simulink model "modelh_age"  (R2020b)
settings: Solver=VariableStepAuto  StartTime=0.0  StopTime=10.0  RelTol=1e-3
values from neighbouring files (symbols this model uses):
  alphaH = 1-exp(-1/d_Hj)    [parameters.m]
  alphaI = 1-exp(-d_Is)    [parameters.m]
  alphaJ = 1-exp(-1/d_J)    [parameters.m]
  gammaA = 1-exp(-1/d_Ia)    [parameters.m]
  gammaH = 1-exp(-1/d_Hr)    [parameters.m]
  gammaZ = 1-exp(-1/d_Iz)    [parameters.m]
  p_d_mu = 0.49    [parameters.m]
  p_d_sd = 0.1    [parameters.m]
  p_h = 0.055    [parameters.m]
  p_j_mu = 0.23    [parameters.m]
  p_j_sd = 0.1    [parameters.m]
  p_s_h = 0.99    [parameters.m]
  p_s_l = 0.5    [parameters.m]
  psi = 1-exp(-1/d_Ip)    [parameters.m]
  r_beta_h = 0.99    [parameters.m]
  r_beta_l = 0.4    [parameters.m]
  r_c_h = 0.5    [parameters.m]
  r_c_l = 0.01    [parameters.m]
  sigma = 1 - exp(-1/d_E)    [parameters.m]
settings Model: Creator=vikroe  LastModifiedBy=vikroe

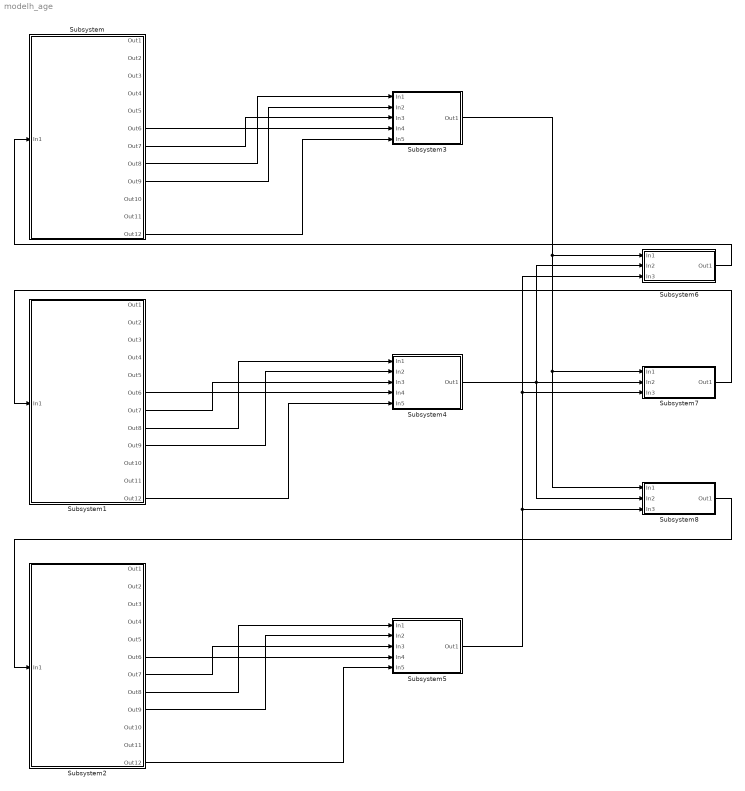
== system modelh_age ==
  Subsystem : Subsystem
  Subsystem1 : Subsystem
  Subsystem2 : Subsystem
  Subsystem3 : Subsystem
  Subsystem4 : Subsystem
  Subsystem5 : Subsystem
  Subsystem6 : Subsystem
  Subsystem7 : Subsystem
  Subsystem8 : Subsystem
  wires:
  Subsystem/12(Out12) -> Subsystem3/5(In5)
  Subsystem/8(Out8) -> Subsystem3/1(In1)
  Subsystem/9(Out9) -> Subsystem3/2(In2)
  Subsystem/7(Out7) -> Subsystem3/3(In3)
  Subsystem/6(Out6) -> Subsystem3/4(In4)
  Subsystem1/6(Out6) -> Subsystem4/4(In4)
  Subsystem1/8(Out8) -> Subsystem4/1(In1)
  Subsystem1/7(Out7) -> Subsystem4/3(In3)
  Subsystem1/9(Out9) -> Subsystem4/2(In2)
  Subsystem1/12(Out12) -> Subsystem4/5(In5)
  Subsystem2/6(Out6) -> Subsystem5/4(In4)
  Subsystem2/8(Out8) -> Subsystem5/1(In1)
  Subsystem2/7(Out7) -> Subsystem5/3(In3)
  Subsystem2/9(Out9) -> Subsystem5/2(In2)
  Subsystem2/12(Out12) -> Subsystem5/5(In5)
  Subsystem3/1(Out1) -> Subsystem6/1(In1), Subsystem7/1(In1), Subsystem8/1(In1)
  Subsystem4/1(Out1) -> Subsystem8/2(In2), Subsystem6/2(In2), Subsystem7/2(In2)
  Subsystem5/1(Out1) -> Subsystem8/3(In3), Subsystem7/3(In3), Subsystem6/3(In3)
  Subsystem6/1(Out1) -> Subsystem/1(In1)
  Subsystem7/1(Out1) -> Subsystem1/1(In1)
  Subsystem8/1(Out1) -> Subsystem2/1(In1)

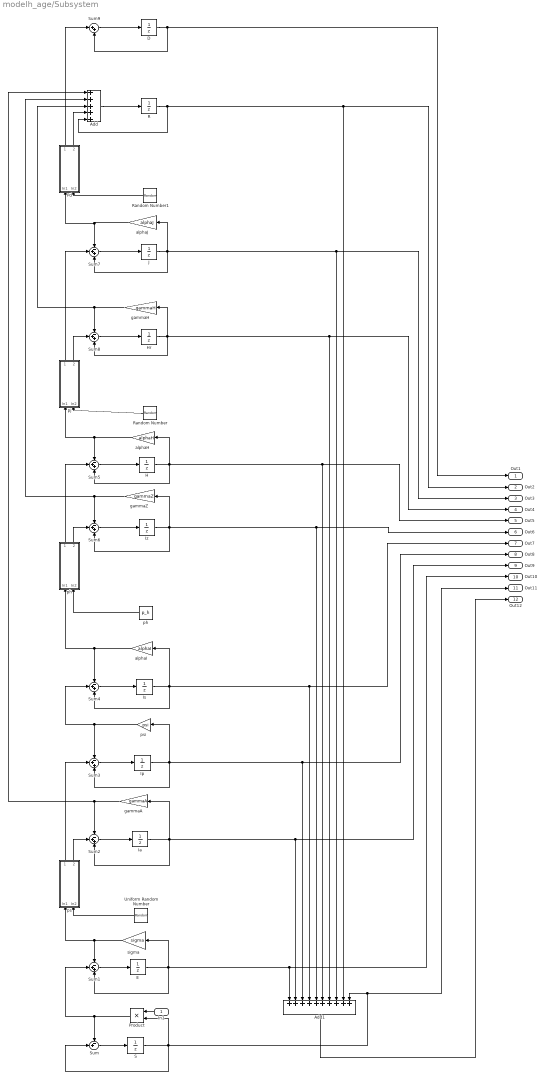
== system modelh_age/Subsystem ==
  In1 : Inport
  Add : Sum  Inputs=+++++
  Add1 : Sum  Inputs=++++++++++
  D : UnitDelay  SampleTime=-1  HasFrameUpgradeWarning=on
  E : UnitDelay  InitialCondition=10000  SampleTime=-1  HasFrameUpgradeWarning=on
  H : UnitDelay  InitialCondition=5000  SampleTime=-1  HasFrameUpgradeWarning=on
  Hr : UnitDelay  InitialCondition=5000  SampleTime=-1  HasFrameUpgradeWarning=on
  Ia : UnitDelay  InitialCondition=5000  SampleTime=-1  HasFrameUpgradeWarning=on
  Ip : UnitDelay  InitialCondition=5000  SampleTime=-1  HasFrameUpgradeWarning=on
  Is : UnitDelay  InitialCondition=5000  SampleTime=-1  HasFrameUpgradeWarning=on
  Iz : UnitDelay  InitialCondition=5000  SampleTime=-1  HasFrameUpgradeWarning=on
  J : UnitDelay  InitialCondition=5000  SampleTime=-1  HasFrameUpgradeWarning=on
  Pd : Subsystem
  Product : Product
  R : UnitDelay  InitialCondition=5000  SampleTime=-1  HasFrameUpgradeWarning=on
  Random Number : RandomNumber  Mean=p_j_mu  Variance=p_j_sd  SampleTime=0.1
  Random Number1 : RandomNumber  Mean=p_d_mu  Variance=p_d_sd  SampleTime=0.1
  S : UnitDelay  InitialCondition=5000000  SampleTime=-1  HasFrameUpgradeWarning=on
  Sum : Sum  Inputs=-+|
  Sum{1..8} (8 alike) : Sum  Inputs=-++
  Sum9 : Sum  Inputs=|++
  Uniform Random Number : UniformRandomNumber  Minimum=p_s_l  Maximum=p_s_h  SampleTime=0.1
  alphaH : Gain  Gain=alphaH
  alphaI : Gain  Gain=alphaI
  alphaJ : Gain  Gain=alphaJ
  gammaA : Gain  Gain=gammaA
  gammaH : Gain  Gain=gammaH
  gammaZ : Gain  Gain=gammaZ
  ph : Subsystem
  "ph " : Constant  Value=p_h
  pj : Subsystem
  "ps " : Subsystem
  psi : Gain  Gain=psi
  sigma : Gain  Gain=sigma
  Out1 : Outport
  Out2 : Outport  Port=2
  Out3 : Outport  Port=3
  Out4 : Outport  Port=4
  Out5 : Outport  Port=5
  Out6 : Outport  Port=6
  Out7 : Outport  Port=7
  Out8 : Outport  Port=8
  Out9 : Outport  Port=9
  Out10 : Outport  Port=10
  Out11 : Outport  Port=11
  Out12 : Outport  Port=12
  wires:
  Sum5/1 -> H/1
  alphaH/1 -> pj/1(In1), Sum5/1
  gammaH/1 -> Sum8/1, Add/3
  "ph "/1 -> ph/2(In2)
  "ps "/1(Out1) -> Sum3/2
  Uniform Random Number/1 -> "ps "/2(In2)
  J/1 -> Out3/1, Add1/8, alphaJ/1, Sum7/3
  ph/1(Out1) -> Sum5/2
  Iz/1 -> Out6/1, Add1/5, gammaZ/1, Sum6/3
  Ip/1 -> Out8/1, Add1/3, psi/1, Sum3/3
  alphaJ/1 -> Pd/1(In1), Sum7/1
  psi/1 -> Sum4/2, Sum3/1
  Ia/1 -> Out9/1, Add1/2, gammaA/1, Sum2/3
  Sum8/1 -> Hr/1
  Sum6/1 -> Iz/1
  Hr/1 -> Out4/1, Add1/7, gammaH/1, Sum8/3
  gammaA/1 -> Sum2/1, Add/1
  Sum4/1 -> Is/1
  D/1 -> Out1/1, Sum9/2
  pj/1(Out1) -> Sum7/2
  Add1/1 -> Out12/1
  Sum1/1 -> E/1
  R/1 -> Out2/1, Add1/9, Add/5
  E/1 -> Out10/1, Add1/1, sigma/1, Sum1/3
  Sum2/1 -> Ia/1
  pj/2(Out2) -> Sum8/2
  Sum9/1 -> D/1
  Random Number1/1 -> Pd/2(In2)
  H/1 -> Out5/1, Add1/6, alphaH/1, Sum5/3
  sigma/1 -> Sum1/1, "ps "/1(In1)
  Add/1 -> R/1
  gammaZ/1 -> Add/2, Sum6/1
  Sum3/1 -> Ip/1
  Sum/1 -> S/1
  Sum7/1 -> J/1
  Random Number/1 -> pj/2(In2)
  Is/1 -> Out7/1, Add1/4, alphaI/1, Sum4/3
  "ps "/2(Out2) -> Sum2/2
  Pd/1(Out1) -> Sum9/1
  ph/2(Out2) -> Sum6/2
  alphaI/1 -> ph/1(In1), Sum4/1
  Product/1 -> Sum1/2, Sum/1
  Pd/2(Out2) -> Add/4
  S/1 -> Product/2, Out11/1, Add1/10, Sum/2
  In1/1 -> Product/1

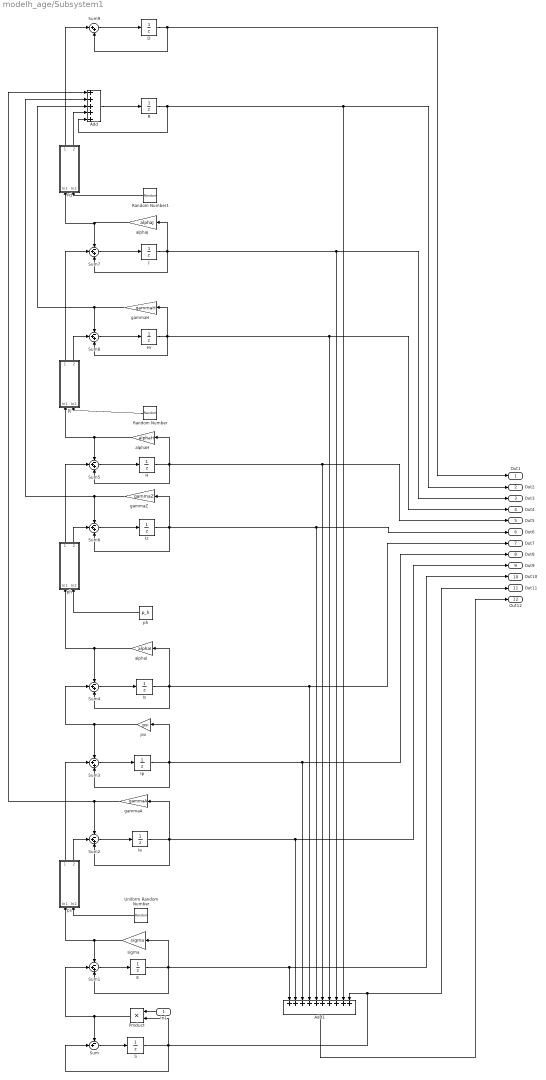
== system modelh_age/Subsystem1 ==
  In1 : Inport
  Add : Sum  Inputs=+++++
  Add1 : Sum  Inputs=++++++++++
  D : UnitDelay  SampleTime=-1  HasFrameUpgradeWarning=on
  E : UnitDelay  InitialCondition=10000  SampleTime=-1  HasFrameUpgradeWarning=on
  H : UnitDelay  InitialCondition=5000  SampleTime=-1  HasFrameUpgradeWarning=on
  Hr : UnitDelay  InitialCondition=5000  SampleTime=-1  HasFrameUpgradeWarning=on
  Ia : UnitDelay  InitialCondition=5000  SampleTime=-1  HasFrameUpgradeWarning=on
  Ip : UnitDelay  InitialCondition=5000  SampleTime=-1  HasFrameUpgradeWarning=on
  Is : UnitDelay  InitialCondition=5000  SampleTime=-1  HasFrameUpgradeWarning=on
  Iz : UnitDelay  InitialCondition=5000  SampleTime=-1  HasFrameUpgradeWarning=on
  J : UnitDelay  InitialCondition=5000  SampleTime=-1  HasFrameUpgradeWarning=on
  Pd : Subsystem
  Product : Product
  R : UnitDelay  InitialCondition=5000  SampleTime=-1  HasFrameUpgradeWarning=on
  Random Number : RandomNumber  Mean=p_j_mu  Variance=p_j_sd  SampleTime=0.1
  Random Number1 : RandomNumber  Mean=p_d_mu  Variance=p_d_sd  SampleTime=0.1
  S : UnitDelay  InitialCondition=5000000  SampleTime=-1  HasFrameUpgradeWarning=on
  Sum : Sum  Inputs=-+|
  Sum{1..8} (8 alike) : Sum  Inputs=-++
  Sum9 : Sum  Inputs=|++
  Uniform Random Number : UniformRandomNumber  Minimum=p_s_l  Maximum=p_s_h  SampleTime=0.1
  alphaH : Gain  Gain=alphaH
  alphaI : Gain  Gain=alphaI
  alphaJ : Gain  Gain=alphaJ
  gammaA : Gain  Gain=gammaA
  gammaH : Gain  Gain=gammaH
  gammaZ : Gain  Gain=gammaZ
  ph : Subsystem
  "ph " : Constant  Value=p_h
  pj : Subsystem
  "ps " : Subsystem
  psi : Gain  Gain=psi
  sigma : Gain  Gain=sigma
  Out1 : Outport
  Out2 : Outport  Port=2
  Out3 : Outport  Port=3
  Out4 : Outport  Port=4
  Out5 : Outport  Port=5
  Out6 : Outport  Port=6
  Out7 : Outport  Port=7
  Out8 : Outport  Port=8
  Out9 : Outport  Port=9
  Out10 : Outport  Port=10
  Out11 : Outport  Port=11
  Out12 : Outport  Port=12
  wires:
  Sum5/1 -> H/1
  alphaH/1 -> pj/1(In1), Sum5/1
  gammaH/1 -> Sum8/1, Add/3
  "ph "/1 -> ph/2(In2)
  "ps "/1(Out1) -> Sum3/2
  Uniform Random Number/1 -> "ps "/2(In2)
  J/1 -> Out3/1, Add1/8, alphaJ/1, Sum7/3
  ph/1(Out1) -> Sum5/2
  Iz/1 -> Out6/1, Add1/5, gammaZ/1, Sum6/3
  Ip/1 -> Out8/1, Add1/3, psi/1, Sum3/3
  alphaJ/1 -> Pd/1(In1), Sum7/1
  psi/1 -> Sum4/2, Sum3/1
  Ia/1 -> Out9/1, Add1/2, gammaA/1, Sum2/3
  Sum8/1 -> Hr/1
  Sum6/1 -> Iz/1
  Hr/1 -> Out4/1, Add1/7, gammaH/1, Sum8/3
  gammaA/1 -> Sum2/1, Add/1
  Sum4/1 -> Is/1
  D/1 -> Out1/1, Sum9/2
  pj/1(Out1) -> Sum7/2
  Add1/1 -> Out12/1
  Sum1/1 -> E/1
  R/1 -> Out2/1, Add1/9, Add/5
  E/1 -> Out10/1, Add1/1, sigma/1, Sum1/3
  Sum2/1 -> Ia/1
  pj/2(Out2) -> Sum8/2
  Sum9/1 -> D/1
  Random Number1/1 -> Pd/2(In2)
  H/1 -> Out5/1, Add1/6, alphaH/1, Sum5/3
  sigma/1 -> Sum1/1, "ps "/1(In1)
  Add/1 -> R/1
  gammaZ/1 -> Add/2, Sum6/1
  Sum3/1 -> Ip/1
  Sum/1 -> S/1
  Sum7/1 -> J/1
  Random Number/1 -> pj/2(In2)
  Is/1 -> Out7/1, Add1/4, alphaI/1, Sum4/3
  "ps "/2(Out2) -> Sum2/2
  Pd/1(Out1) -> Sum9/1
  ph/2(Out2) -> Sum6/2
  alphaI/1 -> ph/1(In1), Sum4/1
  Product/1 -> Sum1/2, Sum/1
  Pd/2(Out2) -> Add/4
  S/1 -> Product/2, Out11/1, Add1/10, Sum/2
  In1/1 -> Product/1

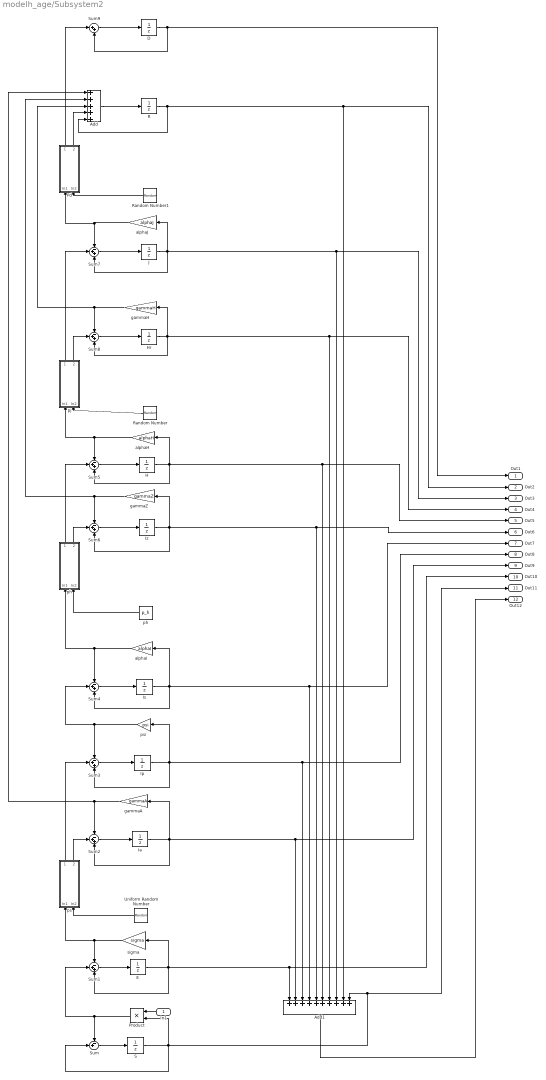
== system modelh_age/Subsystem2 ==
  In1 : Inport
  Add : Sum  Inputs=+++++
  Add1 : Sum  Inputs=++++++++++
  D : UnitDelay  SampleTime=-1  HasFrameUpgradeWarning=on
  E : UnitDelay  InitialCondition=10000  SampleTime=-1  HasFrameUpgradeWarning=on
  H : UnitDelay  InitialCondition=5000  SampleTime=-1  HasFrameUpgradeWarning=on
  Hr : UnitDelay  InitialCondition=5000  SampleTime=-1  HasFrameUpgradeWarning=on
  Ia : UnitDelay  InitialCondition=5000  SampleTime=-1  HasFrameUpgradeWarning=on
  Ip : UnitDelay  InitialCondition=5000  SampleTime=-1  HasFrameUpgradeWarning=on
  Is : UnitDelay  InitialCondition=5000  SampleTime=-1  HasFrameUpgradeWarning=on
  Iz : UnitDelay  InitialCondition=5000  SampleTime=-1  HasFrameUpgradeWarning=on
  J : UnitDelay  InitialCondition=5000  SampleTime=-1  HasFrameUpgradeWarning=on
  Pd : Subsystem
  Product : Product
  R : UnitDelay  InitialCondition=5000  SampleTime=-1  HasFrameUpgradeWarning=on
  Random Number : RandomNumber  Mean=p_j_mu  Variance=p_j_sd  SampleTime=0.1
  Random Number1 : RandomNumber  Mean=p_d_mu  Variance=p_d_sd  SampleTime=0.1
  S : UnitDelay  InitialCondition=5000000  SampleTime=-1  HasFrameUpgradeWarning=on
  Sum : Sum  Inputs=-+|
  Sum{1..8} (8 alike) : Sum  Inputs=-++
  Sum9 : Sum  Inputs=|++
  Uniform Random Number : UniformRandomNumber  Minimum=p_s_l  Maximum=p_s_h  SampleTime=0.1
  alphaH : Gain  Gain=alphaH
  alphaI : Gain  Gain=alphaI
  alphaJ : Gain  Gain=alphaJ
  gammaA : Gain  Gain=gammaA
  gammaH : Gain  Gain=gammaH
  gammaZ : Gain  Gain=gammaZ
  ph : Subsystem
  "ph " : Constant  Value=p_h
  pj : Subsystem
  "ps " : Subsystem
  psi : Gain  Gain=psi
  sigma : Gain  Gain=sigma
  Out1 : Outport
  Out2 : Outport  Port=2
  Out3 : Outport  Port=3
  Out4 : Outport  Port=4
  Out5 : Outport  Port=5
  Out6 : Outport  Port=6
  Out7 : Outport  Port=7
  Out8 : Outport  Port=8
  Out9 : Outport  Port=9
  Out10 : Outport  Port=10
  Out11 : Outport  Port=11
  Out12 : Outport  Port=12
  wires:
  Sum5/1 -> H/1
  alphaH/1 -> pj/1(In1), Sum5/1
  gammaH/1 -> Sum8/1, Add/3
  "ph "/1 -> ph/2(In2)
  "ps "/1(Out1) -> Sum3/2
  Uniform Random Number/1 -> "ps "/2(In2)
  J/1 -> Out3/1, Add1/8, alphaJ/1, Sum7/3
  ph/1(Out1) -> Sum5/2
  Iz/1 -> Out6/1, Add1/5, gammaZ/1, Sum6/3
  Ip/1 -> Out8/1, Add1/3, psi/1, Sum3/3
  alphaJ/1 -> Pd/1(In1), Sum7/1
  psi/1 -> Sum4/2, Sum3/1
  Ia/1 -> Out9/1, Add1/2, gammaA/1, Sum2/3
  Sum8/1 -> Hr/1
  Sum6/1 -> Iz/1
  Hr/1 -> Out4/1, Add1/7, gammaH/1, Sum8/3
  gammaA/1 -> Sum2/1, Add/1
  Sum4/1 -> Is/1
  D/1 -> Out1/1, Sum9/2
  pj/1(Out1) -> Sum7/2
  Add1/1 -> Out12/1
  Sum1/1 -> E/1
  R/1 -> Out2/1, Add1/9, Add/5
  E/1 -> Out10/1, Add1/1, sigma/1, Sum1/3
  Sum2/1 -> Ia/1
  pj/2(Out2) -> Sum8/2
  Sum9/1 -> D/1
  Random Number1/1 -> Pd/2(In2)
  H/1 -> Out5/1, Add1/6, alphaH/1, Sum5/3
  sigma/1 -> Sum1/1, "ps "/1(In1)
  Add/1 -> R/1
  gammaZ/1 -> Add/2, Sum6/1
  Sum3/1 -> Ip/1
  Sum/1 -> S/1
  Sum7/1 -> J/1
  Random Number/1 -> pj/2(In2)
  Is/1 -> Out7/1, Add1/4, alphaI/1, Sum4/3
  "ps "/2(Out2) -> Sum2/2
  Pd/1(Out1) -> Sum9/1
  ph/2(Out2) -> Sum6/2
  alphaI/1 -> ph/1(In1), Sum4/1
  Product/1 -> Sum1/2, Sum/1
  Pd/2(Out2) -> Add/4
  S/1 -> Product/2, Out11/1, Add1/10, Sum/2
  In1/1 -> Product/1

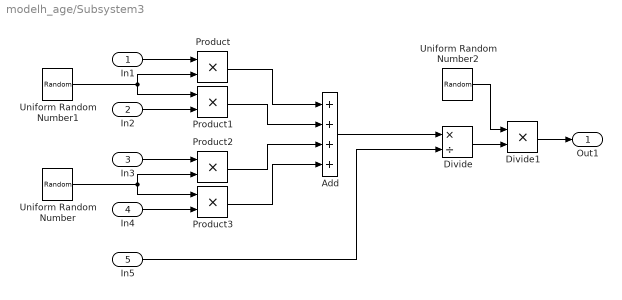
== system modelh_age/Subsystem3 ==
  In1 : Inport
  In2 : Inport  Port=2
  In3 : Inport  Port=3
  In4 : Inport  Port=4
  In5 : Inport  Port=5
  Add : Sum  Inputs=++++
  Divide : Product  Inputs=*/
  Divide1 : Product  Inputs=**
  Product{,1..3} (4 alike) : Product
  Uniform Random Number : UniformRandomNumber  Minimum=r_c_l  Maximum=r_c_h  SampleTime=0.1
  Uniform Random Number1 : UniformRandomNumber  Minimum=r_beta_l  Maximum=r_beta_h  SampleTime=0.1
  Uniform Random Number2 : UniformRandomNumber  SampleTime=0.1
  Out1 : Outport
  wires:
  In1/1 -> Product/1
  In2/1 -> Product1/2
  In3/1 -> Product2/1
  In4/1 -> Product3/2
  Uniform Random Number/1 -> Product3/1, Product2/2
  Uniform Random Number1/1 -> Product1/1, Product/2
  Product1/1 -> Add/2
  Product2/1 -> Add/3
  Product3/1 -> Add/4
  Product/1 -> Add/1
  Add/1 -> Divide/1
  In5/1 -> Divide/2
  Divide/1 -> Divide1/2
  Divide1/1 -> Out1/1
  Uniform Random Number2/1 -> Divide1/1

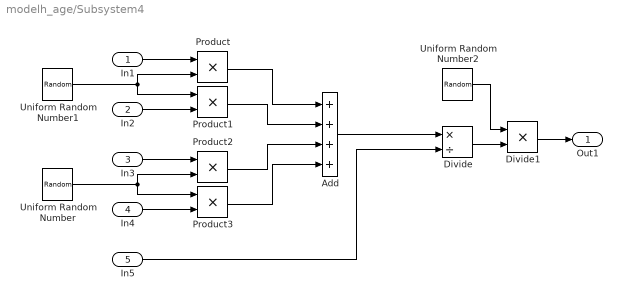
== system modelh_age/Subsystem4 ==
  In1 : Inport
  In2 : Inport  Port=2
  In3 : Inport  Port=3
  In4 : Inport  Port=4
  In5 : Inport  Port=5
  Add : Sum  Inputs=++++
  Divide : Product  Inputs=*/
  Divide1 : Product  Inputs=**
  Product{,1..3} (4 alike) : Product
  Uniform Random Number : UniformRandomNumber  Minimum=r_c_l  Maximum=r_c_h  SampleTime=0.1
  Uniform Random Number1 : UniformRandomNumber  Minimum=r_beta_l  Maximum=r_beta_h  SampleTime=0.1
  Uniform Random Number2 : UniformRandomNumber  SampleTime=0.1
  Out1 : Outport
  wires:
  In3/1 -> Product2/1
  In1/1 -> Product/1
  Divide1/1 -> Out1/1
  Product/1 -> Add/1
  Product3/1 -> Add/4
  Divide/1 -> Divide1/2
  Uniform Random Number/1 -> Product3/1, Product2/2
  Add/1 -> Divide/1
  In5/1 -> Divide/2
  In4/1 -> Product3/2
  In2/1 -> Product1/2
  Uniform Random Number1/1 -> Product1/1, Product/2
  Product1/1 -> Add/2
  Uniform Random Number2/1 -> Divide1/1
  Product2/1 -> Add/3

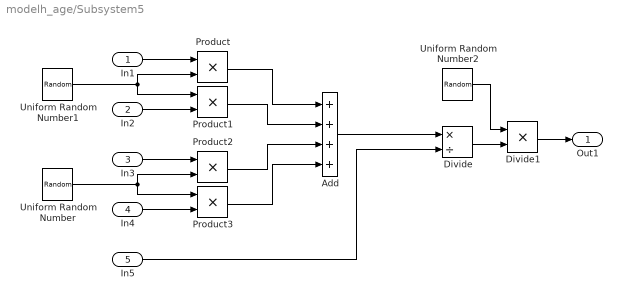
== system modelh_age/Subsystem5 ==
  In1 : Inport
  In2 : Inport  Port=2
  In3 : Inport  Port=3
  In4 : Inport  Port=4
  In5 : Inport  Port=5
  Add : Sum  Inputs=++++
  Divide : Product  Inputs=*/
  Divide1 : Product  Inputs=**
  Product{,1..3} (4 alike) : Product
  Uniform Random Number : UniformRandomNumber  Minimum=r_c_l  Maximum=r_c_h  SampleTime=0.1
  Uniform Random Number1 : UniformRandomNumber  Minimum=r_beta_l  Maximum=r_beta_h  SampleTime=0.1
  Uniform Random Number2 : UniformRandomNumber  SampleTime=0.1
  Out1 : Outport
  wires:
  In3/1 -> Product2/1
  In1/1 -> Product/1
  Divide1/1 -> Out1/1
  Product/1 -> Add/1
  Product3/1 -> Add/4
  Divide/1 -> Divide1/2
  Uniform Random Number/1 -> Product3/1, Product2/2
  Add/1 -> Divide/1
  In5/1 -> Divide/2
  In4/1 -> Product3/2
  In2/1 -> Product1/2
  Uniform Random Number1/1 -> Product1/1, Product/2
  Product1/1 -> Add/2
  Uniform Random Number2/1 -> Divide1/1
  Product2/1 -> Add/3

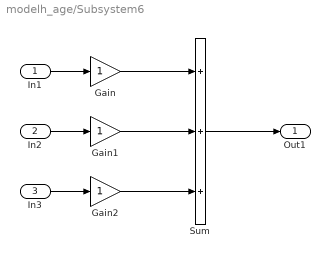
== system modelh_age/Subsystem6 ==
  In1 : Inport
  In2 : Inport  Port=2
  In3 : Inport  Port=3
  Gain : Gain
  Gain1 : Gain
  Gain2 : Gain
  Sum : Sum  Inputs=+++
  Out1 : Outport
  wires:
  In3/1 -> Gain2/1
  In2/1 -> Gain1/1
  In1/1 -> Gain/1
  Gain1/1 -> Sum/2
  Gain/1 -> Sum/1
  Gain2/1 -> Sum/3
  Sum/1 -> Out1/1

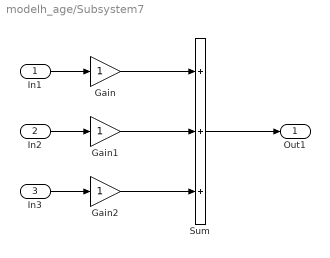
== system modelh_age/Subsystem7 ==
  In1 : Inport
  In2 : Inport  Port=2
  In3 : Inport  Port=3
  Gain : Gain
  Gain1 : Gain
  Gain2 : Gain
  Sum : Sum  Inputs=+++
  Out1 : Outport
  wires:
  In3/1 -> Gain2/1
  In2/1 -> Gain1/1
  In1/1 -> Gain/1
  Gain1/1 -> Sum/2
  Gain/1 -> Sum/1
  Gain2/1 -> Sum/3
  Sum/1 -> Out1/1

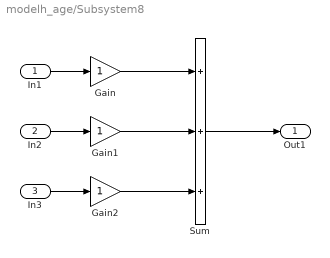
== system modelh_age/Subsystem8 ==
  In1 : Inport
  In2 : Inport  Port=2
  In3 : Inport  Port=3
  Gain : Gain
  Gain1 : Gain
  Gain2 : Gain
  Sum : Sum  Inputs=+++
  Out1 : Outport
  wires:
  In3/1 -> Gain2/1
  In2/1 -> Gain1/1
  In1/1 -> Gain/1
  Gain1/1 -> Sum/2
  Gain/1 -> Sum/1
  Gain2/1 -> Sum/3
  Sum/1 -> Out1/1

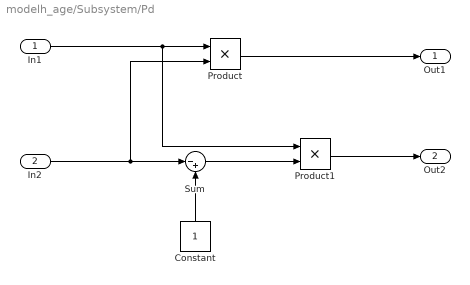
== system modelh_age/Subsystem/Pd ==
  In1 : Inport
  In2 : Inport  Port=2
  Constant : Constant
  Product : Product
  Product1 : Product
  Sum : Sum  Inputs=|-+
  Out1 : Outport
  Out2 : Outport  Port=2
  wires:
  In1/1 -> Product1/1, Product/1
  Product/1 -> Out1/1
  In2/1 -> Sum/1, Product/2
  Constant/1 -> Sum/2
  Sum/1 -> Product1/2
  Product1/1 -> Out2/1

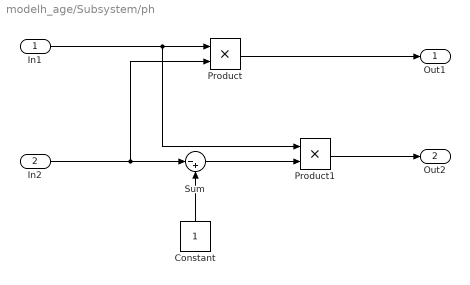
== system modelh_age/Subsystem/ph ==
  In1 : Inport
  In2 : Inport  Port=2
  Constant : Constant
  Product : Product
  Product1 : Product
  Sum : Sum  Inputs=|-+
  Out1 : Outport
  Out2 : Outport  Port=2
  wires:
  In1/1 -> Product1/1, Product/1
  Product/1 -> Out1/1
  In2/1 -> Sum/1, Product/2
  Constant/1 -> Sum/2
  Sum/1 -> Product1/2
  Product1/1 -> Out2/1

== system modelh_age/Subsystem/pj ==
  In1 : Inport
  In2 : Inport  Port=2
  Constant : Constant
  Product : Product
  Product1 : Product
  Sum : Sum  Inputs=|-+
  Out1 : Outport
  Out2 : Outport  Port=2
  wires:
  In1/1 -> Product1/1, Product/1
  Product/1 -> Out1/1
  In2/1 -> Sum/1, Product/2
  Constant/1 -> Sum/2
  Sum/1 -> Product1/2
  Product1/1 -> Out2/1

== system modelh_age/Subsystem/ps  ==
  In1 : Inport
  In2 : Inport  Port=2
  Constant : Constant
  Product : Product
  Product1 : Product
  Sum : Sum  Inputs=|-+
  Out1 : Outport
  Out2 : Outport  Port=2
  wires:
  In1/1 -> Product1/1, Product/1
  Product/1 -> Out1/1
  In2/1 -> Sum/1, Product/2
  Constant/1 -> Sum/2
  Sum/1 -> Product1/2
  Product1/1 -> Out2/1

== system modelh_age/Subsystem1/Pd ==
  In1 : Inport
  In2 : Inport  Port=2
  Constant : Constant
  Product : Product
  Product1 : Product
  Sum : Sum  Inputs=|-+
  Out1 : Outport
  Out2 : Outport  Port=2
  wires:
  In1/1 -> Product1/1, Product/1
  Product/1 -> Out1/1
  In2/1 -> Sum/1, Product/2
  Constant/1 -> Sum/2
  Sum/1 -> Product1/2
  Product1/1 -> Out2/1

== system modelh_age/Subsystem1/ph ==
  In1 : Inport
  In2 : Inport  Port=2
  Constant : Constant
  Product : Product
  Product1 : Product
  Sum : Sum  Inputs=|-+
  Out1 : Outport
  Out2 : Outport  Port=2
  wires:
  In1/1 -> Product1/1, Product/1
  Product/1 -> Out1/1
  In2/1 -> Sum/1, Product/2
  Constant/1 -> Sum/2
  Sum/1 -> Product1/2
  Product1/1 -> Out2/1

== system modelh_age/Subsystem1/pj ==
  In1 : Inport
  In2 : Inport  Port=2
  Constant : Constant
  Product : Product
  Product1 : Product
  Sum : Sum  Inputs=|-+
  Out1 : Outport
  Out2 : Outport  Port=2
  wires:
  In1/1 -> Product1/1, Product/1
  Product/1 -> Out1/1
  In2/1 -> Sum/1, Product/2
  Constant/1 -> Sum/2
  Sum/1 -> Product1/2
  Product1/1 -> Out2/1

== system modelh_age/Subsystem1/ps  ==
  In1 : Inport
  In2 : Inport  Port=2
  Constant : Constant
  Product : Product
  Product1 : Product
  Sum : Sum  Inputs=|-+
  Out1 : Outport
  Out2 : Outport  Port=2
  wires:
  In1/1 -> Product1/1, Product/1
  Product/1 -> Out1/1
  In2/1 -> Sum/1, Product/2
  Constant/1 -> Sum/2
  Sum/1 -> Product1/2
  Product1/1 -> Out2/1

== system modelh_age/Subsystem2/Pd ==
  In1 : Inport
  In2 : Inport  Port=2
  Constant : Constant
  Product : Product
  Product1 : Product
  Sum : Sum  Inputs=|-+
  Out1 : Outport
  Out2 : Outport  Port=2
  wires:
  In1/1 -> Product1/1, Product/1
  Product/1 -> Out1/1
  In2/1 -> Sum/1, Product/2
  Constant/1 -> Sum/2
  Sum/1 -> Product1/2
  Product1/1 -> Out2/1

== system modelh_age/Subsystem2/ph ==
  In1 : Inport
  In2 : Inport  Port=2
  Constant : Constant
  Product : Product
  Product1 : Product
  Sum : Sum  Inputs=|-+
  Out1 : Outport
  Out2 : Outport  Port=2
  wires:
  In1/1 -> Product1/1, Product/1
  Product/1 -> Out1/1
  In2/1 -> Sum/1, Product/2
  Constant/1 -> Sum/2
  Sum/1 -> Product1/2
  Product1/1 -> Out2/1

== system modelh_age/Subsystem2/pj ==
  In1 : Inport
  In2 : Inport  Port=2
  Constant : Constant
  Product : Product
  Product1 : Product
  Sum : Sum  Inputs=|-+
  Out1 : Outport
  Out2 : Outport  Port=2
  wires:
  In1/1 -> Product1/1, Product/1
  Product/1 -> Out1/1
  In2/1 -> Sum/1, Product/2
  Constant/1 -> Sum/2
  Sum/1 -> Product1/2
  Product1/1 -> Out2/1

== system modelh_age/Subsystem2/ps  ==
  In1 : Inport
  In2 : Inport  Port=2
  Constant : Constant
  Product : Product
  Product1 : Product
  Sum : Sum  Inputs=|-+
  Out1 : Outport
  Out2 : Outport  Port=2
  wires:
  In1/1 -> Product1/1, Product/1
  Product/1 -> Out1/1
  In2/1 -> Sum/1, Product/2
  Constant/1 -> Sum/2
  Sum/1 -> Product1/2
  Product1/1 -> Out2/1
